simulink model "ATFIDP_OpenRocket_Integration"  (R2025a)
settings: Solver=ode45  StartTime=0.01  StopTime=1.98  RelTol=1e-3
settings Model: Creator=saipr  LastModifiedBy=saipr

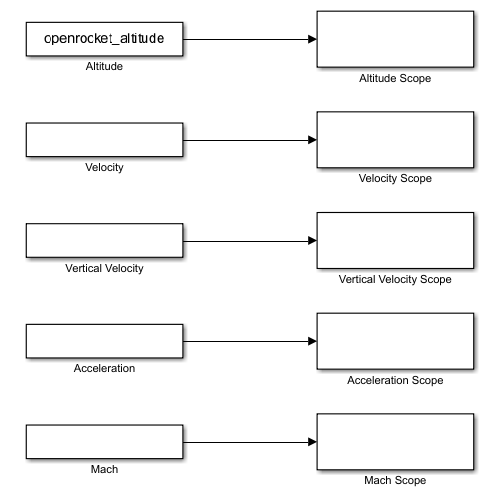
[thumbnail: Simulink's stored preview of the top-level diagram]
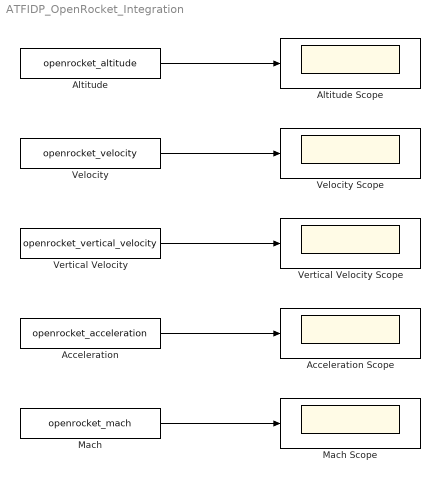
== system ATFIDP_OpenRocket_Integration ==
  Acceleration : FromWorkspace  VariableName=openrocket_acceleration
  Acceleration Scope : Scope
  Altitude : FromWorkspace  VariableName=openrocket_altitude
  Altitude Scope : Scope
  Mach : FromWorkspace  VariableName=openrocket_mach
  Mach Scope : Scope
  Velocity : FromWorkspace  VariableName=openrocket_velocity
  Velocity Scope : Scope
  Vertical Velocity : FromWorkspace  VariableName=openrocket_vertical_velocity
  Vertical Velocity Scope : Scope
  wires:
  Altitude/1 -> Altitude Scope/1
  Velocity/1 -> Velocity Scope/1
  Vertical Velocity/1 -> Vertical Velocity Scope/1
  Acceleration/1 -> Acceleration Scope/1
  Mach/1 -> Mach Scope/1
